simulink model "kyklomaMeRuleBaseKaiFuzzy"  (R2022b)
settings: Solver=ode23tb  StartTime=0.0  StopTime=2  RelTol=1e-5
values from neighbouring files (symbols this model uses):
  Area = 50.6    [FC_Parameters.m]
  B = 0.016    [FC_Parameters.m]
  J_max = 1.5    [FC_Parameters.m]
  ksi4 = -1.93e-4    (= -0.000193)    [FC_Parameters.m]
  N_cells = 35    [FC_Parameters.m]
  PH2 = 1    [FC_Parameters.m]
  PO2 = 0.2095    [FC_Parameters.m]
  R_internal = 0.0003    [FC_Parameters.m]
  T_K = 343    [FC_Parameters.m]
  V_act_const = ksi1 + ksi2*T_K + ksi3*T_K*log(CO2_conc)    [FC_Parameters.m]
undefined symbols (not defined in the file or in its folder): Ion, Lithium, sigbuilder_block
libraries: neural x15, spsParallelRLCBranchLib x4, spsIGBTLib x3, slpidlib x2, spsPWMGeneratorDCDCLib x2, spsBatteryLib x1, spsControlledCurrentSourceLib x1, spsControlledVoltageSourceLib x1, spsCurrentMeasurementLib x1, spsDiodeLib x1, fuzblock x1, rllib x1
(part 2 of 2)

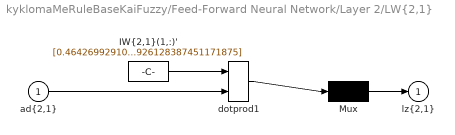
== system kyklomaMeRuleBaseKaiFuzzy/Feed-Forward Neural Network/Layer 2/LW{2,1} ==
  "ad{2,1}" : Inport  PortDimensions=10
      mask Display: e = 0.06;c1 = [120 230 180]/255;c2 = ([120 230 180]+0)/(256+128);c3 = ([120 230 180]+128)/(256+128);patch([0 1 1 0],[0 0 1 1],c1);patch([0 1 1 1-e 1-e 0+e],[0 0 1 1-e 0+e 0+e],c2);patch([0 0 1 1-e 0+e 0+e],[0 1 1 1-e 1-e 0+e],c3);plot([0 1 1 0 0],[0 0 1 1 0]);
  "IW{2,1}(1,:)'" : Constant  Value=[0.464269929100584677339469408252625726163387298583984375;1.41095287486027753942607887438498437404632568359375;-0.05762370826899554376865353333414532244205474853515625;0.1723571936251834524345127874767058528959751129150390625;-0.186522517599133408339184825308620929718017578125;0.2041590907907042673485875639016740024089813232421875;0.68226085738100528121918841861770488321781158447265625;2.475532205435325039388771983794867992401123046875;1.749370360633508258985102656879462301731109619140625;-2.916649438879218347864252791623584926128387451171875]
      mask Display: e = 0.06;c1 = [120 150 230]/255;c2 = ([120 150 230]+0)/383;c3 = ([120 150 230]+128)/383;patch([0 1 1 0],[0 0 1 1],c1);patch([0 1 1 1-e 1-e 0+e],[0 0 1 1-e 0+e 0+e],c2);patch([0 0 1 1-e 0+e 0+e],[0 1 1 1-e 1-e 0+e],c3);plot([0 1 1 0 0],[0 0 1 1 0]);disp('weights');
  Mux : Mux  Inputs=1
      mask Display: e = 0.06;c1 = [120 150 230]/255;c2 = ([120 150 230]+0)/383;c3 = ([120 150 230]+128)/383;patch([0 1 1 0],[0 0 1 1],c1);patch([0 1 1 1-e 1-e 0+e],[0 0 1 1-e 0+e 0+e],c2);patch([0 0 1 1-e 0+e 0+e],[0 1 1 1-e 1-e 0+e],c3);plot([0 1 1 0 0],[0 0 1 1 0]);disp('Mux');
  dotprod1 : neural/Weight Functions/dotprod
  "lz{2,1}" : Outport
      mask Display: e = 0.06;c1 = [120 230 180]/255;c2 = ([120 230 180]+0)/(256+128);c3 = ([120 230 180]+128)/(256+128);patch([0 1 1 0],[0 0 1 1],c1);patch([0 1 1 1-e 1-e 0+e],[0 0 1 1-e 0+e 0+e],c2);patch([0 0 1 1-e 0+e 0+e],[0 1 1 1-e 1-e 0+e],c3);plot([0 1 1 0 0],[0 0 1 1 0]);
  wires:
  "IW{2,1}(1,:)'"/1 -> dotprod1/1
  "ad{2,1}"/1 -> dotprod1/2
  dotprod1/1 -> Mux/1
  Mux/1 -> "lz{2,1}"/1

== matlab function kyklomaMeRuleBaseKaiFuzzy/MATLAB Function1 ==
  data: I_load input; obs output; SOC input; V_bus input
function obs = normalize_inputs(I_load, SOC, V_bus)
    % Κανονικοποίηση εισόδων για το RL Agent
    % Είσοδοι: I_load (A), SOC (%), V_bus (V)
    % Έξοδος: obs [3x1] κανονικοποιημένο
    
    I_load_norm = I_load / 15;              % max = 15A
    SOC_norm    = (SOC - 20) / 60;         % SOC από 20% έως 80%
    V_bus_norm  = V_bus / 48;              % V_bus γύρω από 48V
    
    % Κλιπάρισμα στο [0,1]
    I_load_norm = max(0, min(1, I_load_norm));
    SOC_norm    = max(0, min(1, SOC_norm));
    V_bus_norm  = max(0, min(1.5, V_bus_norm)); % επιτρέπουμε λίγο πάνω από 48V
    
    obs = [I_load_norm; SOC_norm; V_bus_norm]; % έξοδος [3x1]
end

== matlab function kyklomaMeRuleBaseKaiFuzzy/MATLAB Function ==
  data: I_load input; I_fc_ref output; SOC input; V_fc input
function I_fc_ref = rule_based_controller(I_load, SOC, V_fc)
    % --- Παράμετροι Συστήματος ---
    V_bus = 48;             % Σταθερή τάση εξόδου (DC Bus)
    P_fc_max = 1800;        % Μέγιστη ισχύς FC σε Watts[cite: 1]
    P_fc_min = 200;         % Ελάχιστη ισχύς λειτουργίας (idle)[cite: 1]
    P_charge = 400;         % Ισχύς που δεσμεύεται για φόρτιση μπαταρίας[cite: 1]

    % Μετατροπή ρεύματος φορτίου σε ισχύ (P = V * I)
    P_load = I_load * V_bus;

    % Όρια SOC μπαταρίας (Στόχος: διατήρηση γύρω στο 60%)
    SOC_min = 55;
    SOC_max = 65;

    % --- STATE MACHINE (Υπολογισμός Ζητούμενης Ισχύος) ---
    if SOC < SOC_min
        % Mode 1: Φόρτιση Μπαταρίας
        P_req = P_load + P_charge;
        P_fc_ref = min(P_req, P_fc_max); % Προστασία μέγιστης ισχύος[cite: 1]

    elseif SOC > SOC_max
        % Mode 2: Αποφόρτιση Μπαταρίας
        if P_load > P_fc_min + P_charge
            P_fc_ref = P_load - P_charge;
        else
            P_fc_ref = P_fc_min;
        end

    else
        % Mode 3: Load Following (Κανονική λειτουργία 55% - 65%)
        if P_load < P_fc_min
            P_fc_ref = P_fc_min;
        elseif P_load > P_fc_max
            P_fc_ref = P_fc_max;
        else
            P_fc_ref = P_load;
        end
    end

    % --- ΕΞΟΔΟΣ ΡΕΥΜΑΤΟΣ ---
    % Μετατροπή της ζητούμενης ισχύος σε ζητούμενο ρεύμα για την FC (I = P / V)
    if V_fc > 5
        I_fc_ref = P_fc_ref / V_fc;
    else
        I_fc_ref = 0;
    end
end

== matlab function kyklomaMeRuleBaseKaiFuzzy/MATLAB Function2 ==
  data: a input; I_fc_ref output
function I_fc_ref = action_to_current(a)
    I_fc_max = 75.9;
    I_fc_min = 4.9;    % ελάχιστο = P_fc_min/V_fc = 200W/41V
    I_fc_ref = I_fc_min + 0.5*(a+1)*(I_fc_max - I_fc_min);
    I_fc_ref = max(I_fc_min, min(I_fc_max, I_fc_ref));
end

== matlab function kyklomaMeRuleBaseKaiFuzzy/MATLAB Function3 ==
  data: I_load input; SOC input; I_fc input; V_bus input; H2_gs input; reward output
function reward = compute_reward(I_load, SOC, I_fc, V_bus, H2_gs)

    V_bus_ref  = 48;
    V_fc       = 41;
    H2_max_gs  = 75.9 * 0.0003654;
    
    % Ιδανικό ρεύμα για το φορτίο
    P_load     = I_load * V_bus_ref;
    I_fc_ideal = P_load / V_fc;
    
    % 1. Ακολουθία φορτίου (40%)
    r_track = -abs(I_fc - I_fc_ideal) / 75.9;
    
    % 2. Τάση 47-49V (40%)
    if V_bus > 10
        v_error = abs(V_bus - V_bus_ref) / V_bus_ref;
        r_vbus  = -(v_error^2) * 10;
        
        if V_bus < 47
            penalty_v = -5.0;      % κάτω από 47V
        elseif V_bus > 49
            penalty_v = -3.0;      % πάνω από 49V
        else
            penalty_v = 0;         % μέσα στο 47-49V ✅
        end
    else
        r_vbus    = 0;
        penalty_v = 0;
    end
    
    % 3. Κατανάλωση H2 (20%)
    % Τιμωρεί μόνο αν καταναλώνει παραπάνω από το ιδανικό
    I_excess  = max(0, I_fc - I_fc_ideal);
    H2_excess = I_excess * 0.0003654;
    r_h2      = -(H2_excess / H2_max_gs);
    
    % Συνολικό reward
    reward = 0.40*r_track + 0.40*r_vbus + 0.20*r_h2 + penalty_v;
end
